simulink model "PIDTu4_25"  (Simulink 5.0)
settings: Solver=ode45  StartTime=0.0  StopTime=10.0  RelTol=1e-3
libraries: simulink_extras x2
settings Model: LastModifiedBy=ThinkPad

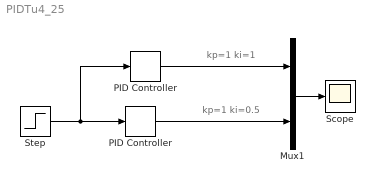
== system PIDTu4_25 ==
  note: kp=1 ki=1
  note: kp=1 ki=0.5
  Mux1 : Mux  Inputs=2
  PID Controller : simulink_extras/Additional Linear/PID Controller  P=1  I=1  D=0
  "PID Controller " : simulink_extras/Additional Linear/PID Controller  P=1  I=0.5  D=0
  Scope : Scope
      settings: YMin=0  YMax=10  SaveName=PIDtu4_25  DataFormat=Array  MaxDataPoints=500000
  Step : Step  SampleTime=0
  wires:
  PID Controller/1 -> Mux1/1
  Step/1 -> "PID Controller "/1, PID Controller/1
  Mux1/1 -> Scope/1
  "PID Controller "/1 -> Mux1/2
